simulink model "resistiveNetwork"  (R2013a)
settings: Solver=ode45  StartTime=0.0  StopTime=9  RelTol=1e-3
libraries: powerlib x11, powerlib_meascontrol x4
settings Model: Creator=DELLPC  LastModifiedBy=hp

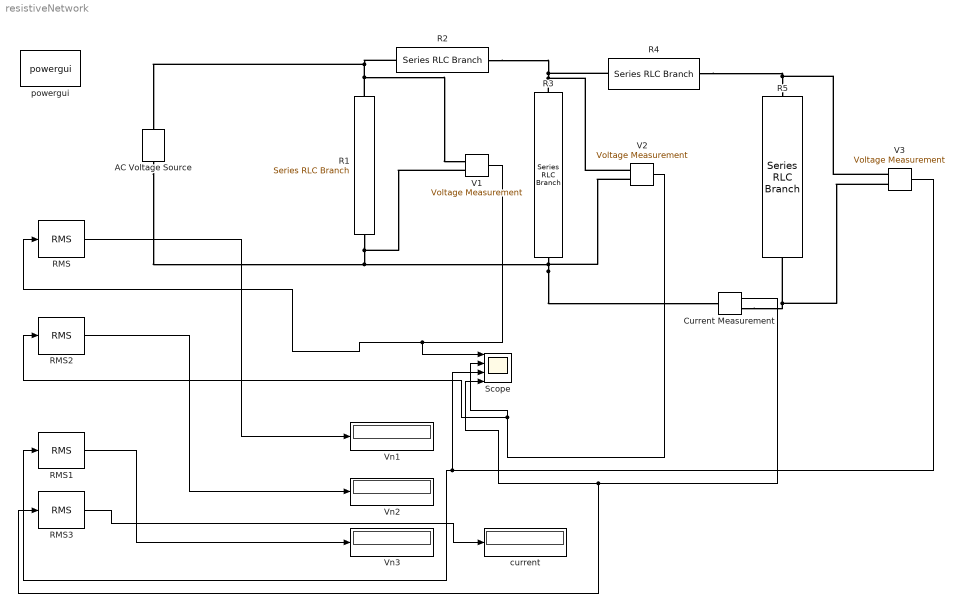
== system resistiveNetwork ==
  AC Voltage Source : powerlib/Electrical Sources/AC Voltage Source  Amplitude=120  Phase=0  Frequency=0.2  SampleTime=0  Measurements=None
  Current Measurement : powerlib/Measurements/Current Measurement  PhasorSimulation=off  OutputType=Complex  PSBequivalent=0
  R1 : powerlib/Elements/Series RLC Branch  LConnTagsString=__new0  RConnTagsString=__new0  BranchType=R  Resistance=20  Inductance=1e-3  SetiL0=off  InitialCurrent=0  Capacitance=1e-6  Setx0=off  InitialVoltage=0  Measurements=None
  R2 : powerlib/Elements/Series RLC Branch  LConnTagsString=__new0  RConnTagsString=__new0  BranchType=R  Resistance=20  Inductance=1e-3  SetiL0=off  InitialCurrent=0  Capacitance=1e-6  Setx0=off  InitialVoltage=0  Measurements=None
  R3 : powerlib/Elements/Series RLC Branch  LConnTagsString=__new0  RConnTagsString=__new0  BranchType=R  Resistance=30  Inductance=1e-3  SetiL0=off  InitialCurrent=0  Capacitance=1e-6  Setx0=off  InitialVoltage=0  Measurements=None
  R4 : powerlib/Elements/Series RLC Branch  LConnTagsString=__new0  RConnTagsString=__new0  BranchType=R  Resistance=40  Inductance=1e-3  SetiL0=off  InitialCurrent=0  Capacitance=1e-6  Setx0=off  InitialVoltage=0  Measurements=None
  R5 : powerlib/Elements/Series RLC Branch  LConnTagsString=__new0  RConnTagsString=__new0  BranchType=R  Resistance=40  Inductance=1e-3  SetiL0=off  InitialCurrent=0  Capacitance=1e-6  Setx0=off  InitialVoltage=0  Measurements=None
  RMS{,1..3} (4 alike) : powerlib_meascontrol/Measurements/RMS  TrueRMS=on  Freq=0.2  RMSInit=120  Ts=0
  Scope : Scope  NumInputPorts=4
      settings: YMin=-5~-5~-5~-5  YMax=5~5~5~5  SaveName=ram
  V1 : powerlib/Measurements/Voltage Measurement  PhasorSimulation=off  OutputType=Complex  PSBequivalent=0
  V2 : powerlib/Measurements/Voltage Measurement  PhasorSimulation=off  OutputType=Complex  PSBequivalent=0
  V3 : powerlib/Measurements/Voltage Measurement  PhasorSimulation=off  OutputType=Complex  PSBequivalent=0
  Vn1 : Display
      settings: Decimation=2
  Vn2 : Display
      settings: Decimation=2
  Vn3 : Display
      settings: Decimation=2
  current : Display
      settings: Decimation=2
  powergui : powerlib/powergui  Priority=1  SimulationMode=Continuous  SolverType=Tustin  SampleTime=50e-6  frequency=60  SPID=off  DisableSnubberDevices=off  DisableRonSwitches=off  DisableVfSwitches=off  SwTol=0  Interpol=off  DisplayEquations=off  frequencyindice=0.2  Pbase=100e6  ErrMax=1e-4  Iterations=50  UnitsV=kV  UnitsW=MW  FunctionMessages=off  echomessages=off  HookPort=off  EnableUseOfTLC=off  x0status=blocks  RestoreLinks=warning  ResistiveCurrentMeasurement=off  Frange=[0:2:500]  Ylog=off  Xlog=on  ShowGrid=off  save=off  variable=ZData  ZoomFFT=off  StartTime=0.0  cycles=1  DisplayStyle=1  fundamental=60  FreqAxis=off  MaxFrequency=1000  frequencyindicesteady=1  RmsSteady=1  display=off  Ts=0  methode=off
  wires:
  V1/1 -> RMS/1, Scope/1
  V3/1 -> RMS1/1, Scope/3
  Current Measurement/1 -> RMS3/1, Scope/4
  V2/1 -> Scope/2, RMS2/1
  RMS2/1 -> Vn2/1
  RMS1/1 -> Vn3/1
  RMS3/1 -> current/1
  RMS/1 -> Vn1/1
  connections:
  R4/LConn1 -- V3/LConn1 -- R5/LConn1
  R4/RConn1 -- R3/LConn1 -- V2/LConn1 -- R2/LConn1
  R2/RConn1 -- V1/LConn1 -- R1/LConn1 -- AC Voltage Source/RConn1
  R3/RConn1 -- AC Voltage Source/LConn1 -- V1/LConn2 -- R1/RConn1 -- V2/LConn2 -- Current Measurement/LConn1
  Current Measurement/RConn1 -- V3/LConn2 -- R5/RConn1
